simulink model "ClosedLoopSystem_PID_Exp"  (R2021a)
settings: Solver=FixedStepAuto  StartTime=0.0  StopTime=tf_raspi  RelTol=1e-3  EnableMultiTasking=on
undefined symbols (not defined in the file or in its folder): ref_angle, tf_raspi, ts_raspi
libraries: simulink x1
settings Model: DataDictionary=sys_PID_data.sldd  Creator=tshintai  LastModifiedBy=tshintai
settings SolverCC: PositivePriorityOrder=on
settings OptimizationCC: EnhancedBackFolding=on  PassReuseOutputArgsAs=Individual arguments  ZeroExternalMemoryAtStartup=off  ZeroInternalMemoryAtStartup=off  MaxStackSize=64  OptimizeBlockOrder=speed  DifferentSizesBufferReuse=on  OptimizationCustomize=off  EfficientTunableParamExpr=on
settings DebuggingCC: ParameterTunabilityLossMsg=error
settings HardwareCC: ProdBitPerPointer=32  ProdBitPerSizeT=32  ProdBitPerPtrDiffT=32  ProdLargestAtomicInteger=Long  ProdLargestAtomicFloat=Double  ProdWordSize=32  ProdLongLongMode=on  ProdHWDeviceType=ARM Compatible->ARM Cortex
settings RTWCC: SystemTargetFile=ert.tlc  HardwareBoard=Raspberry Pi  TLCOptions="-aInlineSetEventsForThisBaseRateFcn=TLC_FALSE -aSuppressMultiTaskScheduler=TLC_FALSE  -aRateBasedStepFcn=0"  TemplateMakefile=ert_default_tmf  Toolchain=GNU GCC Embedded Linux  BuildConfiguration=Faster Runs
settings CodeAppCC: ForceParamTrailComments=on  IgnoreCustomStorageClasses=off  OperatorAnnotations=on  SimulinkDataObjDesc=on  SFDataObjDesc=on  InsertBlockDesc=on
settings ERTTargetCC: SupportVariableSizeSignals=on  ExtModeTransport=2  ExtModeStaticAlloc=on  ExtModeMexFile=ext_xcp  ExtModeIntrfLevel=Level2 - Open

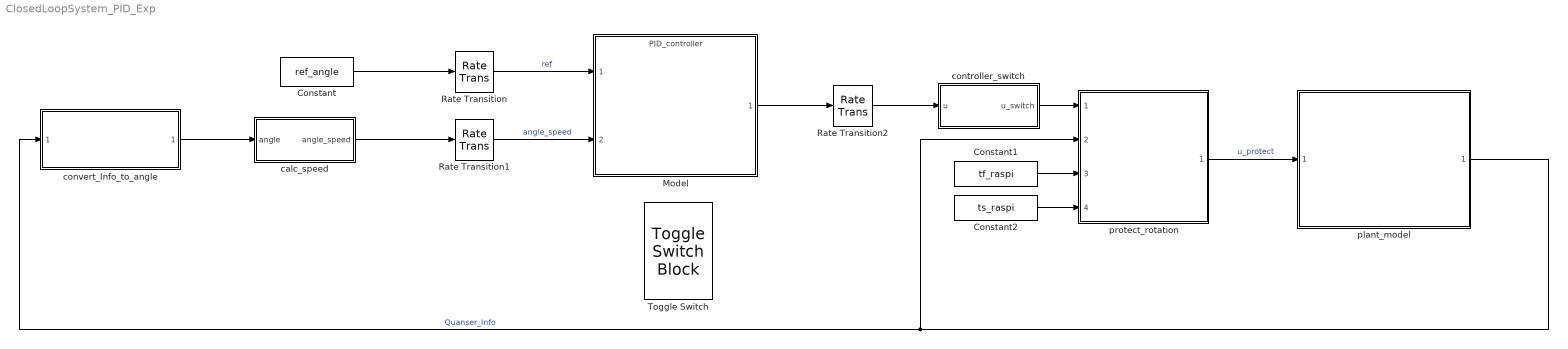
== system ClosedLoopSystem_PID_Exp ==
  Constant : Constant  Value=ref_angle
  Constant1 : Constant  Value=tf_raspi
  Constant2 : Constant  Value=ts_raspi
  Model : ModelReference  ModelNameDialog=PID_controller.slx  SimulationMode=Normal  ModelReferenceVersion=1.54
  Rate Transition : RateTransition  OutPortSampleTime=ts_PID
  Rate Transition1 : RateTransition  OutPortSampleTime=ts_PID
  Rate Transition2 : RateTransition  OutPortSampleTime=ts_raspi
  Toggle Switch : ToggleSwitchBlock
      settings: Values={{'Off', 'On'}, [0 1]}
  calc_speed : Subsystem
  controller_switch : Subsystem
  convert_Info_to_angle : Subsystem  ReferencedSubsystem=convert_Info_to_angle
  plant_model : Subsystem  ReferencedSubsystem=raspi_Quanser
  protect_rotation : Subsystem  ReferencedSubsystem=protect_rotation
  wires:
  Constant1/1 -> protect_rotation/3
  protect_rotation/1 -> plant_model/1  "u_protect"
  Constant2/1 -> protect_rotation/4
  Rate Transition2/1 -> controller_switch/1(u)
  plant_model/1 -> protect_rotation/2, convert_Info_to_angle/1  "Quanser_Info"
  Model/1 -> Rate Transition2/1
  Rate Transition/1 -> Model/1  "ref"
  Rate Transition1/1 -> Model/2  "angle_speed"
  Constant/1 -> Rate Transition/1
  convert_Info_to_angle/1 -> calc_speed/1(angle)
  calc_speed/1(angle_speed) -> Rate Transition1/1
  controller_switch/1(u_switch) -> protect_rotation/1

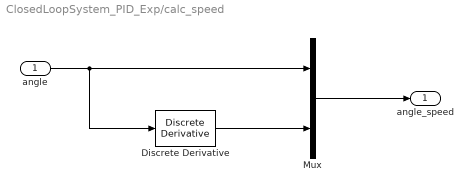
== system ClosedLoopSystem_PID_Exp/calc_speed ==
  angle : Inport
  Discrete Derivative : simulink/Discrete/Discrete Derivative  gainval=1.0  ICPrevScaledInput=0.0  OutMin=[]  OutMax=[]  OutDataType=fixdt(1, 16)  OutScaling=2^-10  DoSatur=off
  Mux : Mux  Inputs=2
  angle_speed : Outport
  wires:
  Mux/1 -> angle_speed/1
  angle/1 -> Discrete Derivative/1, Mux/1
  Discrete Derivative/1 -> Mux/2

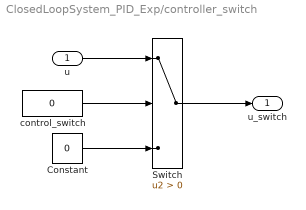
== system ClosedLoopSystem_PID_Exp/controller_switch ==
  u : Inport
  Constant : Constant  Value=0
  Switch : Switch  Criteria=u2 > Threshold
  control_switch : Constant  Value=0  OutDataTypeStr=boolean
  u_switch : Outport
  wires:
  u/1 -> Switch/1
  control_switch/1 -> Switch/2
  Constant/1 -> Switch/3
  Switch/1 -> u_switch/1
